simulink model "simulink_robo_motores"  (R2014a)
settings: Solver=ode45  StartTime=0.0  StopTime=1  RelTol=1e-3
values from neighbouring files (symbols this model uses):
  a = 1    [simula_robo_thiago.m]
  b = 0.1    [simula_robo.m]    (also in simula_robo_thiago.m)
  Ic = 1    [simula_robo_thiago.m]
  Kd = 0    [simula_robo.m]    (also in simula_robo_thiago.m)
  Ki = 10.0    (= 10)    [simula_robo.m]    (also in simula_robo_thiago.m = 0)
  Kp = 5.0    (= 5)    [simula_robo.m]    (also in simula_robo_thiago.m = 50)
  m = 100    [simula_robo_thiago.m]
  r = 0.07    [simula_robo.m]    (also in simula_robo_thiago.m)
libraries: simulink x2
settings Model: Creator=Thiago Lobo  LastModifiedBy=Thiago Lobo

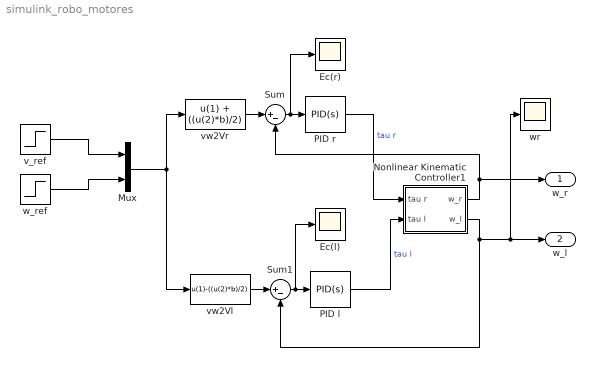
== system simulink_robo_motores ==
  Ec(l) : Scope
      settings: SaveName=ScopeData7
  Ec(r) : Scope
      settings: SaveName=ScopeData6
  Mux : Mux  Inputs=2
  Nonlinear Kinematic Controller1 : Subsystem
  PID l : simulink/Continuous/PID Controller  Controller=PID  TimeDomain=Continuous-time  SampleTime=1  IntegratorMethod=Forward Euler  FilterMethod=Forward Euler  Form=Parallel  P=Kp  I=Ki  D=Kd  N=100  InitialConditionSource=internal  InitialConditionForIntegrator=0  InitialConditionForFilter=0  ExternalReset=none  LimitOutput=off  UpperSaturationLimit=inf  LowerSaturationLimit=-inf  LinearizeAsGain=on  AntiWindupMode=none  Kb=1  TrackingMode=off  Kt=1  PParamMin=[]  PParamMax=[]  IParamMin=[]  IParamMax=[]  DParamMin=[]  DParamMax=[]  NParamMin=[]  NParamMax=[]  KbParamMin=[]  KbParamMax=[]  KtParamMin=[]  KtParamMax=[]  POutMin=[]  POutMax=[]  IOutMin=[]  IOutMax=[]  DOutMin=[]  DOutMax=[]  NOutMin=[]  NOutMax=[]  KbOutMin=[]  KbOutMax=[]  KtOutMin=[]  KtOutMax=[]  IntegratorOutMin=[]  IntegratorOutMax=[]  FilterOutMin=[]  FilterOutMax=[]  SumOutMin=[]  SumOutMax=[]  SumI1OutMin=[]  SumI1OutMax=[]  SumI2OutMin=[]  SumI2OutMax=[]  SumI3OutMin=[]  SumI3OutMax=[]  SumDOutMin=[]  SumDOutMax=[]  SaturationOutMin=[]  SaturationOutMax=[]  IntegratorContinuousStateAttributes=''  IntegratorStateMustResolveToSignalObject=off  IntegratorRTWStateStorageClass=Auto  FilterContinuousStateAttributes=''  FilterStateMustResolveToSignalObject=off  FilterRTWStateStorageClass=Auto
  PID r : simulink/Continuous/PID Controller  Controller=PID  TimeDomain=Continuous-time  SampleTime=1  IntegratorMethod=Forward Euler  FilterMethod=Forward Euler  Form=Parallel  P=Kp  I=Ki  D=Kd  N=100  InitialConditionSource=internal  InitialConditionForIntegrator=0  InitialConditionForFilter=0  ExternalReset=none  LimitOutput=off  UpperSaturationLimit=inf  LowerSaturationLimit=-inf  LinearizeAsGain=on  AntiWindupMode=none  Kb=1  TrackingMode=off  Kt=1  PParamMin=[]  PParamMax=[]  IParamMin=[]  IParamMax=[]  DParamMin=[]  DParamMax=[]  NParamMin=[]  NParamMax=[]  KbParamMin=[]  KbParamMax=[]  KtParamMin=[]  KtParamMax=[]  POutMin=[]  POutMax=[]  IOutMin=[]  IOutMax=[]  DOutMin=[]  DOutMax=[]  NOutMin=[]  NOutMax=[]  KbOutMin=[]  KbOutMax=[]  KtOutMin=[]  KtOutMax=[]  IntegratorOutMin=[]  IntegratorOutMax=[]  FilterOutMin=[]  FilterOutMax=[]  SumOutMin=[]  SumOutMax=[]  SumI1OutMin=[]  SumI1OutMax=[]  SumI2OutMin=[]  SumI2OutMax=[]  SumI3OutMin=[]  SumI3OutMax=[]  SumDOutMin=[]  SumDOutMax=[]  SaturationOutMin=[]  SaturationOutMax=[]  IntegratorContinuousStateAttributes=''  IntegratorStateMustResolveToSignalObject=off  IntegratorRTWStateStorageClass=Auto  FilterContinuousStateAttributes=''  FilterStateMustResolveToSignalObject=off  FilterRTWStateStorageClass=Auto
  Sum : Sum  Inputs=|+-
  Sum1 : Sum  Inputs=|+-
  v_ref : Step  Before=1  SampleTime=0
  vw2Vl : Fcn  Expr=u(1)-((u(2)*b)/2)
  vw2Vr : Fcn  Expr=u(1) + ((u(2)*b)/2)
  w_ref : Step  After=0  SampleTime=0
  wr : Scope
      settings: SaveName=ScopeData3
  w_r : Outport
  w_l : Outport  Port=2
  wires:
  Mux/1 -> vw2Vr/1, vw2Vl/1
  PID r/1 -> Nonlinear Kinematic Controller1/1(tau r)  "tau r"
  Sum/1 -> Ec(r)/1, PID r/1
  PID l/1 -> Nonlinear Kinematic Controller1/2(tau l)  "tau l"
  vw2Vl/1 -> Sum1/1
  Sum1/1 -> Ec(l)/1, PID l/1
  Nonlinear Kinematic Controller1/1(w_r) -> w_r/1, Sum/2
  Nonlinear Kinematic Controller1/2(w_l) -> wr/1, w_l/1, Sum1/2
  v_ref/1 -> Mux/1
  w_ref/1 -> Mux/2
  vw2Vr/1 -> Sum/1

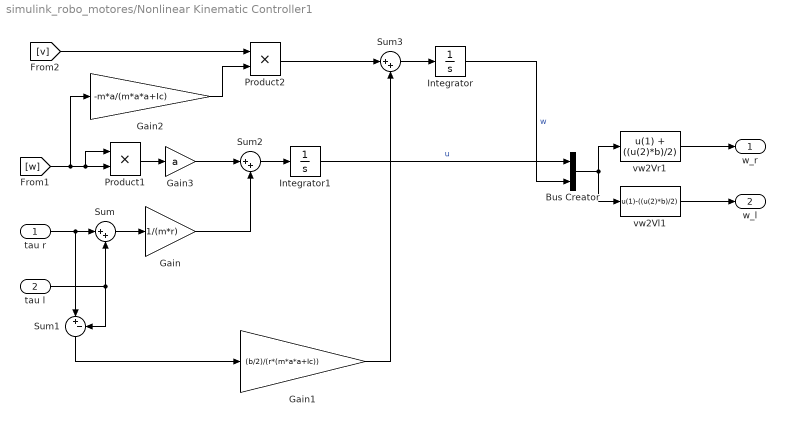
== system simulink_robo_motores/Nonlinear Kinematic Controller1 ==
  tau r : Inport
  tau l : Inport  Port=2
  Bus Creator : BusCreator  Inputs=2
  Gain : Gain  Gain=1/(m*r)
  Gain1 : Gain  Gain=(b/2)/(r*(m*a*a+Ic))
  Gain2 : Gain  Gain=-m*a/(m*a*a+Ic)
  Gain3 : Gain  Gain=a
  Integrator : Integrator
  Integrator1 : Integrator
  Product1 : Product
  Product2 : Product
  Sum : Sum  Inputs=|++
  Sum1 : Sum  Inputs=|+-
  Sum2 : Sum  Inputs=|++
  Sum3 : Sum  Inputs=|++
  vw2Vl1 : Fcn  Expr=u(1)-((u(2)*b)/2)
  vw2Vr1 : Fcn  Expr=u(1) + ((u(2)*b)/2)
  w_r : Outport
  w_l : Outport  Port=2
  wires:
  tau r/1 -> Sum1/1, Sum/1
  tau l/1 -> Sum/2, Sum1/2
  Sum/1 -> Gain/1
  Product1/1 -> Gain3/1
  Gain3/1 -> Sum2/1
  Gain/1 -> Sum2/2
  Sum1/1 -> Gain1/1
  [w] -> Gain2/1, Product1/1, Product1/2
  [v] -> Product2/1
  Gain2/1 -> Product2/2
  Product2/1 -> Sum3/1
  Gain1/1 -> Sum3/2
  Integrator1/1 -> Bus Creator/1  "u"
  Sum2/1 -> Integrator1/1
  Sum3/1 -> Integrator/1
  Integrator/1 -> Bus Creator/2  "w"
  vw2Vr1/1 -> w_r/1
  vw2Vl1/1 -> w_l/1
  Bus Creator/1 -> vw2Vl1/1, vw2Vr1/1
